simulink model "ostim_proses_LinearClosedLoopSimulink"  (R2021b)
settings: Solver=FixedStepAuto  StartTime=0.0  StopTime=50000  FixedStep=1  RelTol=1e-3
values from neighbouring files (symbols this model uses):
  K1 = (cp_fluid*(Ths-Tc1s))/(m_tank1*cp_tank)    [LinearModelParameters.m]
  K10 = ((-URes*A_res)/(mh*cp_fluid)) + ((-UT1*AT1_surf)/(mh*cp_fluid)) + ((-UT2*AT2_surf)/(mh*cp_fluid))    (= -0.0383842150256)    [LinearModelParameters.m]
  K11 = (-URes*A_res)/(mh*cp_fluid)    (= -6.62699306817e-05)    [LinearModelParameters.m]
  K12 = (-UT1*AT1_surf)/(mh*cp_fluid)    (= -0.0246188373131)    [LinearModelParameters.m]
  K13 = (-UT2*AT2_surf)/(mh*cp_fluid)    (= -0.0136991077818)    [LinearModelParameters.m]
  K2 = (mp1*cp_fluid)/(m_tank1*cp_tank)    (= 0.002)    [LinearModelParameters.m]
  K3 = (-UT1*AT1_surf)/(m_tank1*cp_tank)    (= -8.88740027002e-05)    [LinearModelParameters.m]
  K4 = -K3    (= 8.88740027002e-05)    [LinearModelParameters.m]
  K5 = (cp_fluid*(Ths-Tc2s))/(m_tank2*cp_tank)    [LinearModelParameters.m]
  K6 = mp2*cp_fluid/(m_tank2*cp_tank)    (= 0.00344017094017)    [LinearModelParameters.m]
  K7 = (-UT2*AT2_surf)/(m_tank2*cp_tank)    (= -0.000105670468146)    [LinearModelParameters.m]
  K8 = -K7    (= 0.000105670468146)    [LinearModelParameters.m]
  K9 = 1/(mh*cp_fluid)    (= 6.62699306817e-05)    [LinearModelParameters.m]
  T1s = T1(end)    [LinearModelParameters.m]
  T2s = T2(end)    [LinearModelParameters.m]
  Ths = Th(end)    [LinearModelParameters.m]
settings Model: Creator=ismt  LastModifiedBy=ismt

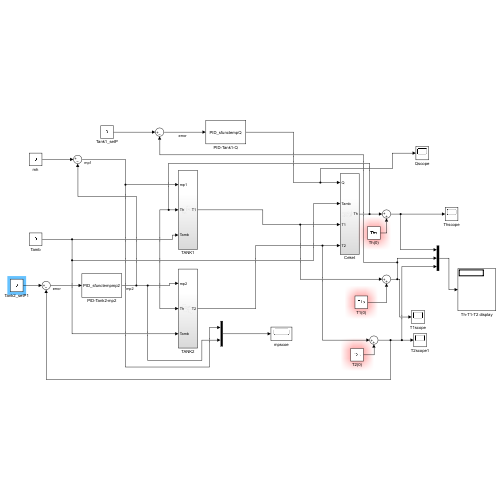
[thumbnail: Simulink's stored preview of the top-level diagram]
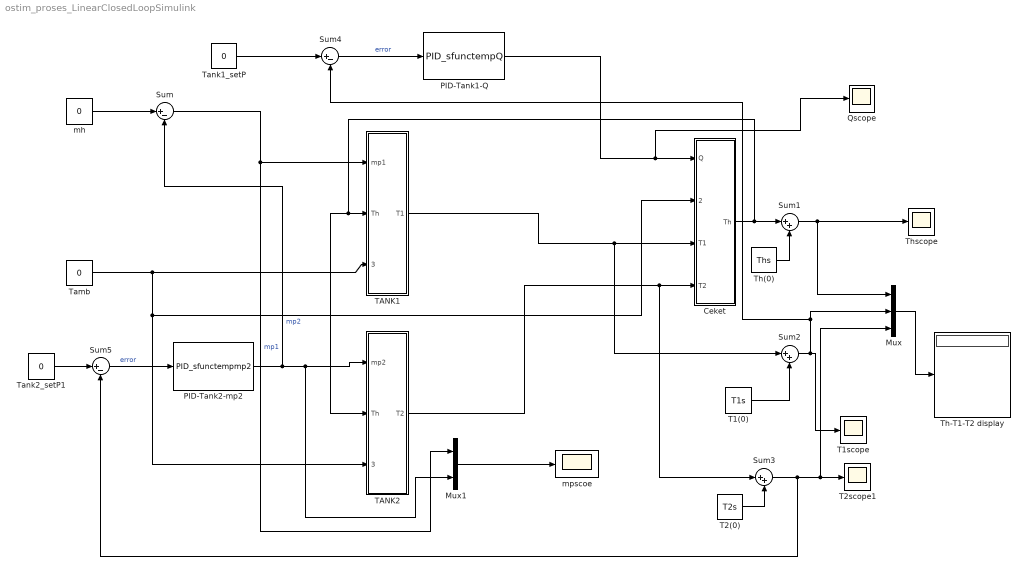
== system ostim_proses_LinearClosedLoopSimulink ==
  Ceket : Subsystem
  Mux : Mux  Inputs=3
  Mux1 : Mux  Inputs=2
  PID-Tank1-Q : S-Function  FunctionName=PID_sfunctempQ  Parameters=KC,TI,TD  SFunctionDeploymentMode=off  EnableBusSupport=off  mask{KC=3, TI=15, TD=3}
  PID-Tank2-mp2 : S-Function  FunctionName=PID_sfunctempmp2  Parameters=KC,TI,TD  SFunctionDeploymentMode=off  EnableBusSupport=off  mask{KC=1, TI=10000, TD=10}
  Qscope : Scope
  Sum : Sum  Inputs=|+-
  Sum1 : Sum  Inputs=|++
  Sum2 : Sum  Inputs=|++
  Sum3 : Sum  Inputs=|++
  Sum4 : Sum  Inputs=|+-
  Sum5 : Sum  Inputs=|+-
  T1(0) : Constant  Value=T1s
  T1scope : Scope
  T2(0) : Constant  Value=T2s
  T2scope1 : Scope
  TANK1 : Subsystem
  TANK2 : Subsystem
  Tamb : Constant  Value=0
  Tank1_setP : Constant  Value=0
  Tank2_setP1 : Constant  Value=0
  Th(0) : Constant  Value=Ths
  Th-T1-T2 display : Display
  Thscope : Scope
  mh : Constant  Value=0
  mpscoe : Scope
  wires:
  Tamb/1 -> TANK1/3(Tamb), Ceket/2(Tamb), TANK2/3(Tamb)
  TANK1/1(T1) -> Sum2/1, Ceket/3(T1)
  mh/1 -> Sum/1
  Ceket/1(Th) -> Sum1/1, TANK1/2(Th), TANK2/2(Th)
  Sum1/1 -> Mux/1, Thscope/1
  TANK2/1(T2) -> Sum3/1, Ceket/4(T2)
  Sum2/1 -> Sum4/2, Mux/2, T1scope/1
  Sum3/1 -> Sum5/2, Mux/3, T2scope1/1
  Mux/1 -> Th-T1-T2 display/1
  Th(0)/1 -> Sum1/2
  T1(0)/1 -> Sum2/2
  T2(0)/1 -> Sum3/2
  Tank1_setP/1 -> Sum4/1
  Sum4/1 -> PID-Tank1-Q/1  "error"
  Sum/1 -> Mux1/1, TANK1/1(mp1)  "mp1"
  Tank2_setP1/1 -> Sum5/1
  Sum5/1 -> PID-Tank2-mp2/1  "error"
  PID-Tank2-mp2/1 -> Mux1/2, TANK2/1(mp2), Sum/2  "mp2"
  PID-Tank1-Q/1 -> Qscope/1, Ceket/1(Q)
  Mux1/1 -> mpscoe/1

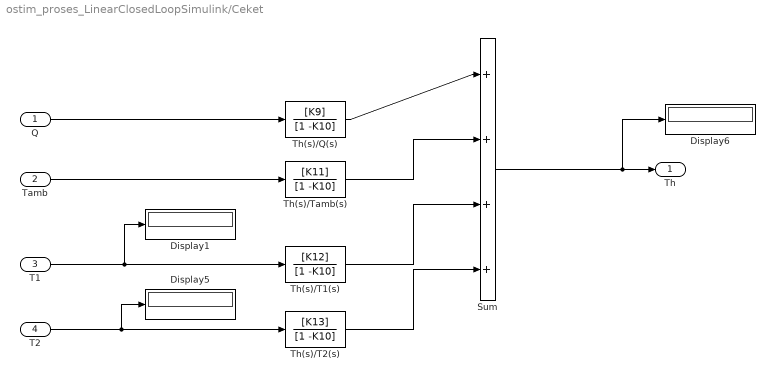
== system ostim_proses_LinearClosedLoopSimulink/Ceket ==
  Q : Inport
  Tamb : Inport  Port=2
  T1 : Inport  Port=3
  T2 : Inport  Port=4
  Display1 : Display
  Display5 : Display
  Display6 : Display
  Sum : Sum  Inputs=|++++
  Th(s)/Q(s) : TransferFcn  Numerator=[K9]  Denominator=[1 -K10]
  Th(s)/T1(s) : TransferFcn  Numerator=[K12]  Denominator=[1 -K10]
  Th(s)/T2(s) : TransferFcn  Numerator=[K13]  Denominator=[1 -K10]
  Th(s)/Tamb(s) : TransferFcn  Numerator=[K11]  Denominator=[1 -K10]
  Th : Outport
  wires:
  Q/1 -> Th(s)/Q(s)/1
  Sum/1 -> Display6/1, Th/1
  T1/1 -> Display1/1, Th(s)/T1(s)/1
  Tamb/1 -> Th(s)/Tamb(s)/1
  T2/1 -> Display5/1, Th(s)/T2(s)/1
  Th(s)/Q(s)/1 -> Sum/1
  Th(s)/Tamb(s)/1 -> Sum/2
  Th(s)/T1(s)/1 -> Sum/3
  Th(s)/T2(s)/1 -> Sum/4

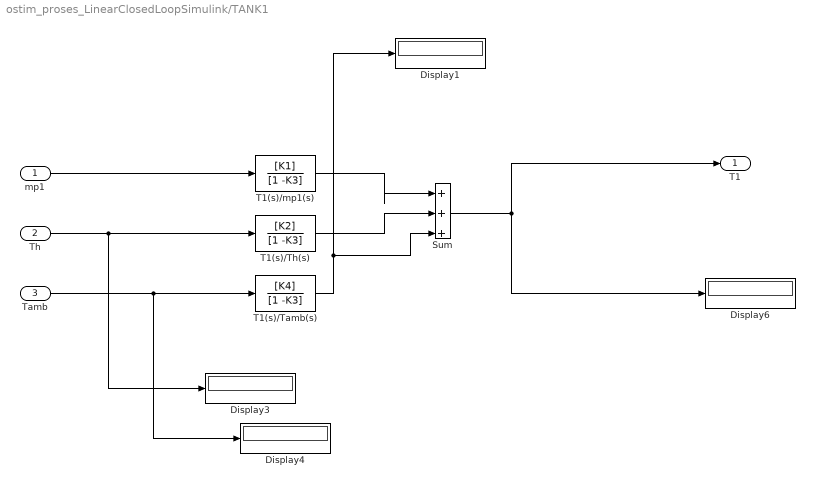
== system ostim_proses_LinearClosedLoopSimulink/TANK1 ==
  mp1 : Inport
  Th : Inport  Port=2
  Tamb : Inport  Port=3
  Display{1,3..4,6} (4 alike) : Display
  Sum : Sum  Inputs=|+++
  T1(s)/Tamb(s) : TransferFcn  Numerator=[K4]  Denominator=[1 -K3]
  T1(s)/Th(s) : TransferFcn  Numerator=[K2]  Denominator=[1 -K3]
  T1(s)/mp1(s) : TransferFcn  Numerator=[K1]  Denominator=[1 -K3]
  T1 : Outport
  wires:
  T1(s)/Tamb(s)/1 -> Sum/3, Display1/1
  mp1/1 -> T1(s)/mp1(s)/1
  Sum/1 -> Display6/1, T1/1
  Th/1 -> Display3/1, T1(s)/Th(s)/1
  Tamb/1 -> Display4/1, T1(s)/Tamb(s)/1
  T1(s)/mp1(s)/1 -> Sum/1
  T1(s)/Th(s)/1 -> Sum/2

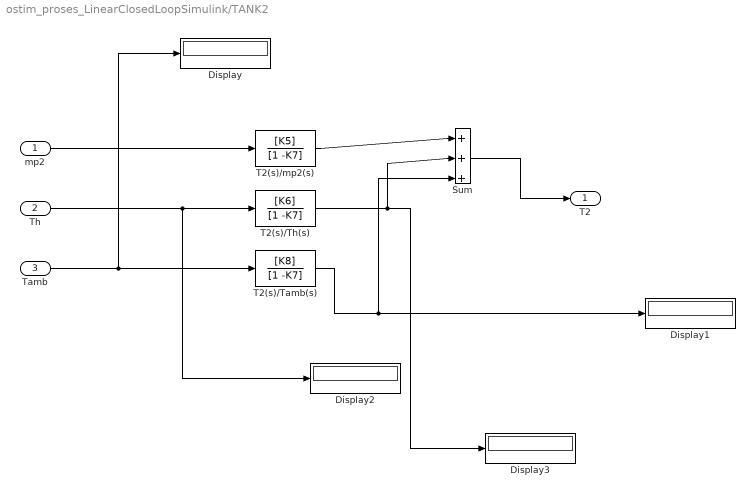
== system ostim_proses_LinearClosedLoopSimulink/TANK2 ==
  mp2 : Inport
  Th : Inport  Port=2
  Tamb : Inport  Port=3
  Display{,1..3} (4 alike) : Display
  Sum : Sum  Inputs=|+++
  T2(s)/Tamb(s) : TransferFcn  Numerator=[K8]  Denominator=[1 -K7]
  T2(s)/Th(s) : TransferFcn  Numerator=[K6]  Denominator=[1 -K7]
  T2(s)/mp2(s) : TransferFcn  Numerator=[K5]  Denominator=[1 -K7]
  T2 : Outport
  wires:
  Tamb/1 -> Display/1, T2(s)/Tamb(s)/1
  Th/1 -> Display2/1, T2(s)/Th(s)/1
  Sum/1 -> T2/1
  mp2/1 -> T2(s)/mp2(s)/1
  T2(s)/Tamb(s)/1 -> Sum/3, Display1/1
  T2(s)/Th(s)/1 -> Sum/2, Display3/1
  T2(s)/mp2(s)/1 -> Sum/1
